simulink model "LowLevelControlPositionMode"  (R2022a)
settings: Solver=ode4  StartTime=0.0  StopTime=Inf  FixedStep=1/500  RelTol=1e-3
undefined symbols (not defined in the file): HIL
libraries: quarc_library x9, simulink x1
settings Model: ExtModeTrigDuration=10000  Creator=fvranes  LastModifiedBy=lgonzalez
settings SolverCC: AlgebraicLoopSolver=TrustRegion
settings DataIOCC: ReturnWorkspaceOutputs=off
settings DebuggingCC: UnderspecifiedInitializationDetection=Classic  MergeDetectMultiDrivingBlocksExec=none  UnconnectedInputMsg=warning  UnconnectedOutputMsg=warning  UnconnectedLineMsg=warning
settings ModelReferenceCC: PropagateSignalLabelsOutOfModel=off
settings SFSimCC: CustomCodeUndefinedFunction=UseInterfaceOnly

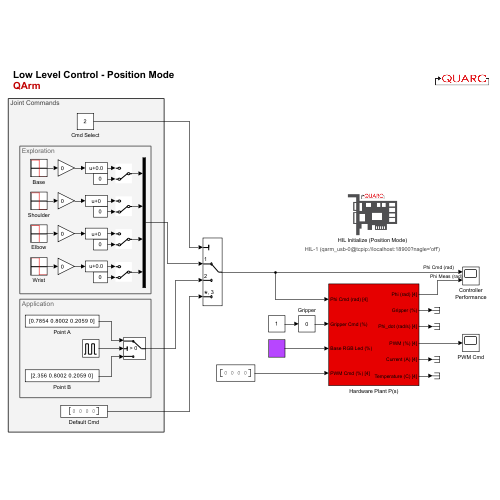
[thumbnail: Simulink's stored preview of the top-level diagram]
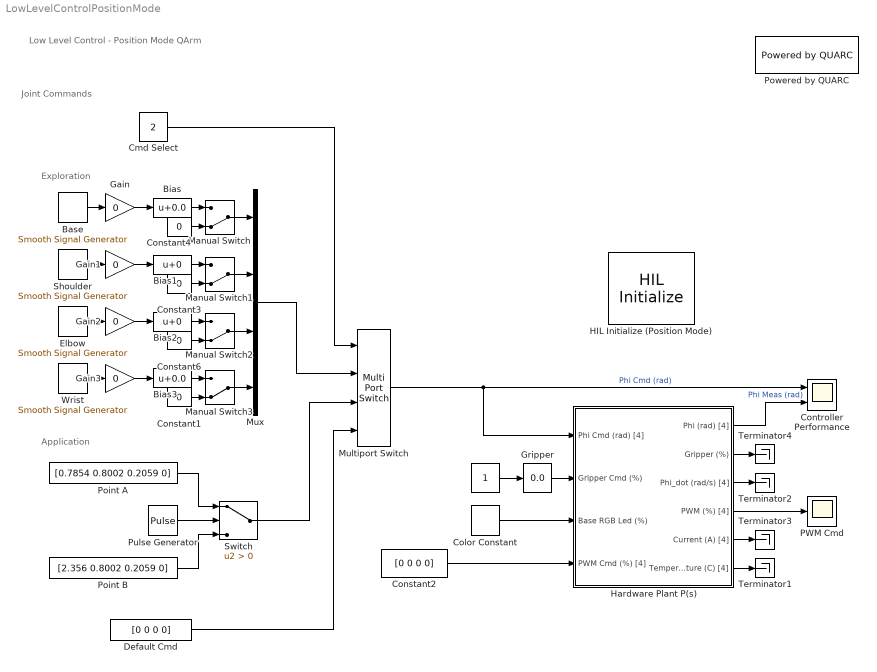
== system LowLevelControlPositionMode ==
  note: Joint Commands
  note: Application
  note: Exploration
  note: Low Level Control - Position Mode
      | QArm
  " " : Constant
  Base : quarc_library/Sources/Signals/Smooth Signal Generator  signal_type=Square  source=Internal (dialog parameters)  amplitude=pi/4  frequency=0.1  initial_phase=0  sample_time=qc_get_step_size  output_cos=off
      settings: SourceProductName=QUARC Targets
  Bias : Bias  Bias=0.0  SaturateOnIntegerOverflow=off
  Bias1 : Bias  SaturateOnIntegerOverflow=off
  Bias2 : Bias  SaturateOnIntegerOverflow=off
  Bias3 : Bias  Bias=0.0  SaturateOnIntegerOverflow=off
  Cmd Select : Constant  Value=2
  Color Constant : quarc_library/Sources/Signals/Color Constant  color=[0.71765 0.27451 1]
      settings: SourceProductName=QUARC Targets
  Constant{1,3..4,6} (4 alike) : Constant  Value=0
  Constant2 : Constant  Value=[0 0 0 0]
  Controller Performance : Scope  NumInputPorts=2
  Default Cmd : Constant  Value=[0 0 0 0]
  Elbow : quarc_library/Sources/Signals/Smooth Signal Generator  signal_type=Square  source=Internal (dialog parameters)  amplitude=pi/4  frequency=0.1  initial_phase=pi  sample_time=qc_get_step_size  output_cos=off
      settings: SourceProductName=QUARC Targets
  Gain{,1..3} (4 alike) : Gain  Gain=0
  Gripper : simulink/Math Operations/Slider Gain  gain=0.0  low=0  high=1
  HIL Initialize (Position Mode) : quarc_library/Data Acquisition/Generic/Configuration/HIL Initialize  object_name=HIL-1  board_type=qarm_usb  board_number=0@tcpip://localhost:18900?nagle='off'  board_options=j0_mode=0;j1_mode=0;j2_mode=0;j3_mode=0;gripper_mode=0;  exclusive=off  active=on  hardware_clocks=[0]  clock_modes=[]  initial_clock_frequencies=[]  set_clock_params_at_start=off  set_clock_params_at_switch_in=off  set_clock_frequencies_at_start=off  set_clock_frequencies_at_switch_in=off  analog_input_channels=[5:9]  analog_input_configurations=[]  analog_input_maximums=[]  analog_input_minimums=[]  set_analog_input_params_at_start=off  set_analog_input_params_at_switch_in=off  analog_output_channels=[]  analog_output_maximums=inf  analog_output_minimums=-inf  initial_analog_outputs=[0]  final_analog_outputs=[0]  watchdog_analog_outputs=[]  set_analog_output_params_at_start=off  set_analog_output_params_at_switch_in=off  set_analog_outputs_at_start=off  set_analog_outputs_at_switch_in=off  set_analog_outputs_at_terminate=off  set_analog_outputs_at_switch_out=off  set_analog_outputs_on_watchdog=off  digital_input_channels=[]  digital_output_channels=[]  digital_output_configuration=[]  initial_digital_outputs=[0]  final_digital_outputs=[0]  watchdog_digital_outputs=[0]  set_digital_output_params_at_start=off  set_digital_output_params_at_switch_in=off  set_digital_outputs_at_start=off  set_digital_outputs_at_switch_in=off  set_digital_outputs_at_terminate=off  set_digital_outputs_at_switch_out=off  set_digital_outputs_on_watchdog=off  encoder_channels=[]  quadrature=[]  encoder_filter_frequency=[]  initial_encoder_counts=[]  set_encoder_params_at_start=off  set_encoder_params_at_switch_in=off  set_encoder_counts_at_start=off  set_encoder_counts_at_switch_in=off  pwm_channels=[]  pwm_modes=[]  pwm_frequency=[]  pwm_configuration=[]  pwm_alignment=[]  pwm_polarity=[]  pwm_leading_deadband=[]  pwm_trailing_deadband=[]  initial_pwm_outputs=[]  final_pwm_outputs=[]  watchdog_pwm_outputs=[]  set_pwm_params_at_start=off  set_pwm_params_at_switch_in=off  set_pwm_outputs_at_start=off  set_pwm_outputs_at_switch_in=off  set_pwm_outputs_at_terminate=off  set_pwm_outputs_at_switch_out=off  set_pwm_outputs_on_watchdog=off  other_output_channels=[1000:1004 11000:11003 11005:11007]  initial_other_outputs=[zeros(1,9), ones(1,3)]  final_other_outputs=[zeros(1,9), ones(1,3)]  watchdog_other_outputs=zeros(1,12)  set_other_outputs_at_start=off  set_other_outputs_at_switch_in=off  set_other_outputs_at_terminate=on  set_other_outputs_at_switch_out=off  set_other_outputs_on_watchdog=off
  Hardware Plant P(s) : Subsystem
  Manual Switch{,1..3} (4 alike) : ManualSwitch  CurrentSetting=0
  Multiport Switch : MultiPortSwitch  SaturateOnIntegerOverflow=off  InputSameDT=off
  Mux : Mux
  PWM Cmd : Scope
  Point A : Constant  Value=[0.7854 0.8002 0.2059 0]
  Point B : Constant  Value=[2.356 0.8002 0.2059 0]
  Powered by QUARC : quarc_library/Logos/Powered by QUARC
  Pulse Generator : DiscretePulseGenerator  PulseType=Time based  Period=10  PulseWidth=50
  Shoulder : quarc_library/Sources/Signals/Smooth Signal Generator  signal_type=Square  source=Internal (dialog parameters)  amplitude=pi/4  frequency=0.1  initial_phase=0  sample_time=qc_get_step_size  output_cos=off
      settings: SourceProductName=QUARC Targets
  Switch : Switch  Criteria=u2 > Threshold  SaturateOnIntegerOverflow=off  InputSameDT=off
  Terminator{1..4} (4 alike) : Terminator
  Wrist : quarc_library/Sources/Signals/Smooth Signal Generator  signal_type=Square  source=Internal (dialog parameters)  amplitude=pi/4  frequency=0.1  initial_phase=0  sample_time=qc_get_step_size  output_cos=off
      settings: SourceProductName=QUARC Targets
  wires:
  Color Constant/1 -> Hardware Plant P(s)/3(Base RGB Led (%))
  Hardware Plant P(s)/6(Temperature (C) [4]) -> Terminator1/1
  Hardware Plant P(s)/3(Phi_dot (rad/s) [4]) -> Terminator2/1
  Hardware Plant P(s)/5(Current (A) [4]) -> Terminator3/1
  Gripper/1 -> Hardware Plant P(s)/2(Gripper Cmd (%))
  Hardware Plant P(s)/2(Gripper (%)) -> Terminator4/1
  Hardware Plant P(s)/4(PWM (%) [4]) -> PWM Cmd/1
  Hardware Plant P(s)/1(Phi (rad) [4]) -> Controller Performance/2  "Phi Meas (rad)"
  Default Cmd/1 -> Multiport Switch/4
  " "/1 -> Gripper/1
  Switch/1 -> Multiport Switch/3
  Pulse Generator/1 -> Switch/2
  Point B/1 -> Switch/3
  Point A/1 -> Switch/1
  Cmd Select/1 -> Multiport Switch/1
  Constant2/1 -> Hardware Plant P(s)/4(PWM Cmd (%) [4])
  Multiport Switch/1 -> Controller Performance/1, Hardware Plant P(s)/1(Phi Cmd (rad) [4])  "Phi Cmd (rad)"
  Gain2/1 -> Bias2/1
  Gain3/1 -> Bias3/1
  Gain/1 -> Bias/1
  Gain1/1 -> Bias1/1
  Base/1 -> Gain/1
  Constant6/1 -> Manual Switch2/2
  Bias2/1 -> Manual Switch2/1
  Bias/1 -> Manual Switch/1
  Manual Switch/1 -> Mux/1
  Bias3/1 -> Manual Switch3/1
  Bias1/1 -> Manual Switch1/1
  Manual Switch1/1 -> Mux/2
  Manual Switch3/1 -> Mux/4
  Elbow/1 -> Gain2/1
  Shoulder/1 -> Gain1/1
  Wrist/1 -> Gain3/1
  Constant3/1 -> Manual Switch1/2
  Constant1/1 -> Manual Switch3/2
  Manual Switch2/1 -> Mux/3
  Constant4/1 -> Manual Switch/2
  Mux/1 -> Multiport Switch/2

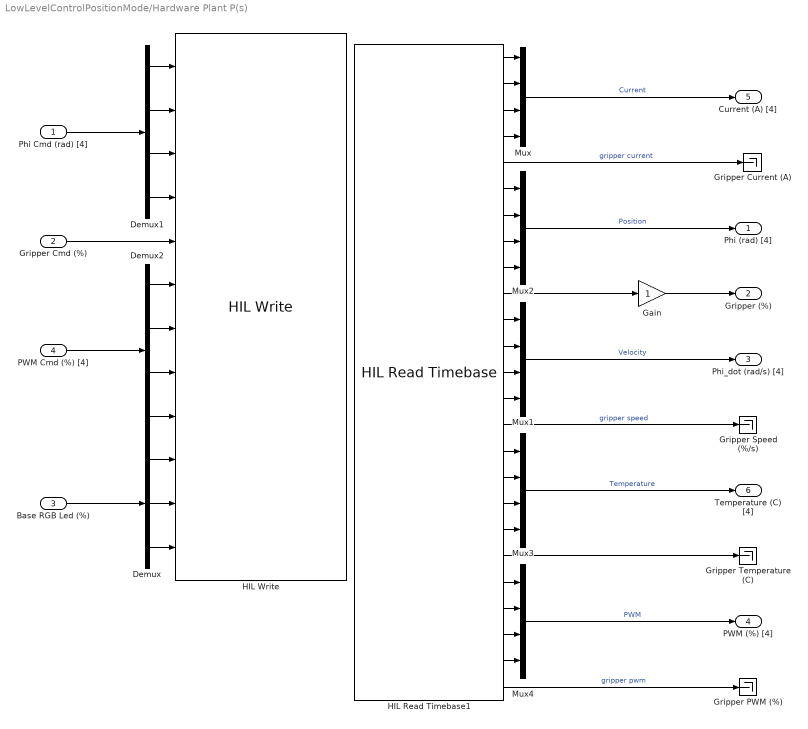
== system LowLevelControlPositionMode/Hardware Plant P(s) ==
  Phi Cmd (rad) [4] : Inport
  Gripper Cmd (%) : Inport  Port=2
  Base RGB Led (%) : Inport  Port=3
  PWM Cmd (%) [4] : Inport  Port=4
  Demux : Demux  Outputs=3
  Demux1 : Demux
  Demux2 : Demux
  Gain : Gain
  Gripper Current (A) : Terminator
  Gripper PWM (%) : Terminator
  Gripper Speed (%/s) : Terminator
  Gripper Temperature (C) : Terminator
  HIL Read Timebase1 : quarc_library/Data Acquisition/Generic/Timebases/HIL Read Timebase  object_name=HIL-1  clock=0  analog_channels=[5:9]  encoder_channels=[]  digital_channels=[]  other_channels=[1000:1004 3000:3004 10000:10004 11000:11004]  active=on  vector_output=off  data_type_mode=Inherit via back propagation  encoder_data_type=double  digital_data_type=boolean  overflow_mode=Synchronize (for simulated cards only)  samples_in_buffer=1
  HIL Write : quarc_library/Data Acquisition/Generic/Immediate I//O/HIL Write  object_name=HIL-1  analog_channels=[]  pwm_channels=[]  digital_channels=[]  other_channels=[1000:1004 11000:11003 11005:11007]  sample_time=-1  active=on  vector_input=off
  Mux{,1..4} (5 alike) : Mux
  Phi (rad) [4] : Outport  VectorParamsAs1DForOutWhenUnconnected=off
  Gripper (%) : Outport  Port=2  VectorParamsAs1DForOutWhenUnconnected=off
  Phi_dot (rad/s) [4] : Outport  Port=3  VectorParamsAs1DForOutWhenUnconnected=off
  PWM (%) [4] : Outport  Port=4  VectorParamsAs1DForOutWhenUnconnected=off
  Current (A) [4] : Outport  Port=5  VectorParamsAs1DForOutWhenUnconnected=off
  Temperature (C) [4] : Outport  Port=6  VectorParamsAs1DForOutWhenUnconnected=off
  wires:
  HIL Read Timebase1/14 -> Mux1/4
  HIL Read Timebase1/9 -> Mux2/4
  HIL Read Timebase1/6 -> Mux2/1
  HIL Read Timebase1/18 -> Mux3/3
  HIL Read Timebase1/8 -> Mux2/3
  HIL Read Timebase1/12 -> Mux1/2
  HIL Read Timebase1/4 -> Mux/4
  HIL Read Timebase1/7 -> Mux2/2
  HIL Read Timebase1/5 -> Gripper Current (A)/1  "gripper current"
  HIL Read Timebase1/15 -> Gripper Speed (%/s)/1  "gripper speed"
  Demux/3 -> HIL Write/12
  HIL Read Timebase1/3 -> Mux/3
  HIL Read Timebase1/17 -> Mux3/2
  HIL Read Timebase1/16 -> Mux3/1
  HIL Read Timebase1/11 -> Mux1/1
  Demux/1 -> HIL Write/10
  HIL Read Timebase1/19 -> Mux3/4
  Demux/2 -> HIL Write/11
  HIL Read Timebase1/13 -> Mux1/3
  HIL Read Timebase1/2 -> Mux/2
  HIL Read Timebase1/1 -> Mux/1
  HIL Read Timebase1/20 -> Gripper Temperature (C)/1
  Mux/1 -> Current (A) [4]/1  "Current"
  Mux1/1 -> Phi_dot (rad/s) [4]/1  "Velocity"
  Mux3/1 -> Temperature (C) [4]/1  "Temperature"
  Base RGB Led (%)/1 -> Demux/1
  Demux1/1 -> HIL Write/1
  Demux1/2 -> HIL Write/2
  Demux1/3 -> HIL Write/3
  Demux1/4 -> HIL Write/4
  Phi Cmd (rad) [4]/1 -> Demux1/1
  PWM Cmd (%) [4]/1 -> Demux2/1
  Demux2/1 -> HIL Write/6
  Demux2/2 -> HIL Write/7
  Demux2/3 -> HIL Write/8
  Demux2/4 -> HIL Write/9
  Mux2/1 -> Phi (rad) [4]/1  "Position"
  HIL Read Timebase1/21 -> Mux4/1
  HIL Read Timebase1/22 -> Mux4/2
  HIL Read Timebase1/23 -> Mux4/3
  HIL Read Timebase1/24 -> Mux4/4
  HIL Read Timebase1/25 -> Gripper PWM (%)/1  "gripper pwm"
  Mux4/1 -> PWM (%) [4]/1  "PWM"
  HIL Read Timebase1/10 -> Gain/1
  Gain/1 -> Gripper (%)/1
  Gripper Cmd (%)/1 -> HIL Write/5
